simulink model "SimBAlink_CL"  (R2017a)
settings: Solver=ode1  StartTime=0.0  StopTime=Inf  FixedStep=0.01  RelTol=1e-3  EnableMultiTasking=on
PreLoadFcn:
  | clear all
  | close all
  | clc
  | 
  | currentFolder = pwd;
  | addpath(genpath(currentFolder));
values from neighbouring files (symbols this model uses):
  ambTemp_K = ambTemp_C + 273.5    [Initialize_Environment.m]    (also in Initialize_Environment_CDTS.m; Initialize_Environment_combined.m)
  Stoptime = 60    [Initialize_Environment.m]    (also in Initialize_Environment_CDTS.m; Initialize_Environment_combined.m; Initialize_Sim.m)
undefined symbols (not defined in the file or in its folder): BATT_ELEC, BATT_OCV, BATT_THERMAL, EM, MC, soc0
libraries: simulink x5
settings Model: Creator=bring  LastModifiedBy=bring
settings DataIOCC: LimitDataPoints=on  SaveFormat=Array  SignalLoggingSaveFormat=ModelDataLogs
settings OptimizationCC: ExpressionDepthLimit=2147483647  LifeSpan=inf
settings DebuggingCC: CheckSSInitialOutputMsg=off  UnderspecifiedInitializationDetection=Classic  MergeDetectMultiDrivingBlocksExec=none  SolverPrmCheckMsg=warning  FcnCallInpInsideContextMsg=warning  StateNameClashWarn=warning  SFUnexpectedBacktrackingDiag=warning  SFNoUnconditionalDefaultTransitionDiag=warning  SFExecutionAtInitializationDiag=none
settings HardwareCC: ProdBitPerPointer=32  ProdBitPerSizeT=32  ProdBitPerPtrDiffT=32  ProdLargestAtomicFloat=None  ProdIntDivRoundTo=Undefined  ProdEndianess=Unspecified  ProdWordSize=32  ProdHWDeviceType=32-bit Generic
settings ModelReferenceCC: PropagateSignalLabelsOutOfModel=off
settings SFSimCC: SimParseCustomCode=off
settings GRTTargetCC: TargetLangStandard=C89/C90 (ANSI)  GeneratePreprocessorConditionals=Disable all  CombineOutputUpdateFcns=off  GRTInterface=on
settings ConfigComp: CovMetricSettings=dw  CovHtmlReporting=on  CovSaveCumulativeToWorkspaceVar=on  CovSaveSingleToWorkspaceVar=on  CovExternalEMLEnable=off  CovSFcnEnable=off

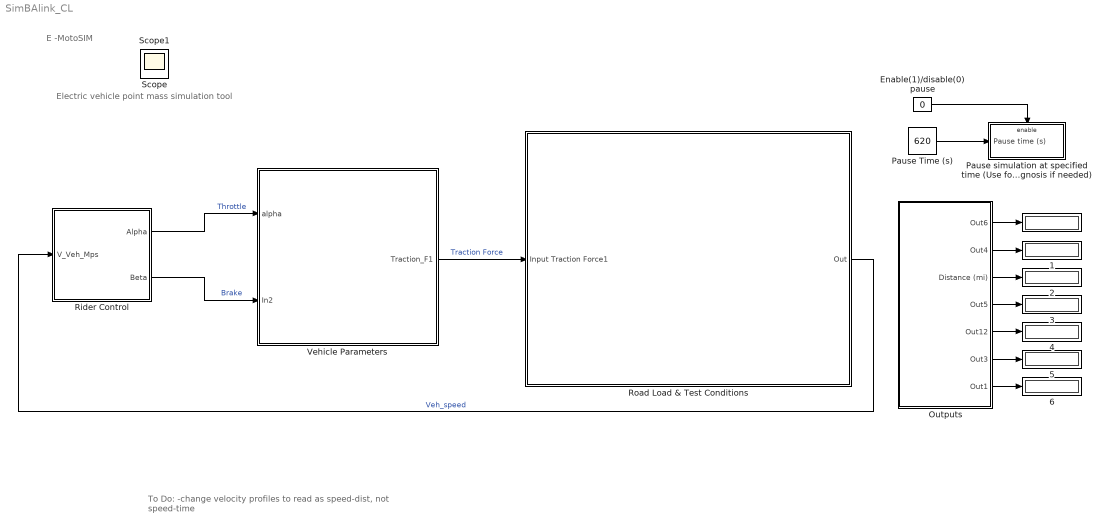
== system SimBAlink_CL ==
  note: To Do:
      | -change velocity profiles to read as speed-dist, not speed-time
  note: Electric vehicle point mass simulation tool
  note: E -MotoSIM
   {,1..6} (7 alike) : Display
  Enable(1)/disable(0) pause : Constant  Value=0
  Outputs : Subsystem  mask(Outputs){}
  Pause Time (s) : Constant  Value=620
  Pause simulation at specified time (Use for diagnosis if needed) : Subsystem
  Rider Control : Subsystem  mask(Driver){kp=1, ki=0.1, kd=0.1}
      mask prompts: kp "Proportional Gain"; ki "Integral Gain"; kd "Derivative Gain"
      mask help: Please select the PID controller gains to improve the tracking response.
      mask Display: image(imread('Images/helmet.jpg'))
  Road Load & Test Conditions : Subsystem  mask(Simulation Setup Options){DRIV_Cycle=US06_Highway_Cycle, rowA=1.13, ambTemp_C=20, soc0=95, Grade_Value=0, Wind_Speed=0, iteration=2, DRIV_acc_flag=off, DRIV_acc_final_v=100}
      mask prompts: DRIV_Cycle "Velocity Profile"; rowA "Air Density (kg.m^3)"; ambTemp_C "Ambient Temperature (C)"; soc0 "Battery Initial SOC (%)"; Grade_Value "Road Grade Climb (deg)"; Wind_Speed "Wind Speed (m/s)"; iteration "Driving Cycle Repetition"; DRIV_acc_flag "Acceleration Test"; DRIV_acc_final_v "Acceleration Test Final Velocity (mph)"
      mask init:
      | Initialize_Environment
      mask TypeOptions DRIV_Cycle: FHDS | FUDS | FUDS_fast | WLTP | US06 | US06_City_Cycle | US06_Highway_Cycle | Artemis_urban | Artemis_extra_urban | Artemis_highway | NEDC | PPIHC_CDTS
      mask Display: image(imread('images/bike.jpg'))
  Vehicle Parameters : Subsystem  mask(Vehicle Setup Options){baseMass=100, TIRE_radius=0.3, CdA=0.38, maxBrakeTorque=2000, FrontSprocket_toothCt=22, RearSprocket_toothCt=54, EM_MC_Selection=emrax268_PM150DZR, regenPct=0, CELL_Selection=LiFePo4_generic, cellSeriesCount=134, cellParallelCount=7, cellCapacity=17.5, ambTemp_C=270}
      mask prompts: baseMass "Vehicle+Rider Base Mass (kg)"; TIRE_radius "Tire Radius (m)"; maxBrakeTorque "Max Brake Torque (Nm)"; FrontSprocket_toothCt "Fr Sprocket Teeth"; RearSprocket_toothCt "Rr Sprocket Teeth"; EM_MC_Selection "Motor-MC Combo"; regenPct "Regen %"; CELL_Selection "Battery Cell Chemistry"; cellSeriesCount "Series Cells"; cellParallelCount "Parallel Cells"; cellCapacity "Cell Capacity (Ah)"; ambTemp_C "Ambient Temperature (C)"
      mask init:
      | Initialize_Vehicle
      mask TypeOptions EM_MC_Selection: emrax268_PM150DZR | ME708_KDS48200e
      mask TypeOptions CELL_Selection: LiFePo4_generic | A123_ANR26650
      mask DialogControl baseMass Tooltip: Vehicle+Rider Base Mass includes all components except EM, MC, and battery pack
      mask Display: image(imread('images/bike_powertrain.jpg'))
  Scope : Scope
  Scope1 : Scope
  wires:
  Road Load & Test Conditions/1(Out) -> Rider Control/1(V_Veh_Mps)  "Veh_speed"
  Rider Control/2(Beta) -> Vehicle Parameters/2(In2)  "Brake"
  Rider Control/1(Alpha) -> Vehicle Parameters/1(alpha)  "Throttle"
  Vehicle Parameters/1(Traction_F1) -> Road Load & Test Conditions/1(Input Traction Force1)  "Traction Force"
  Pause Time (s)/1 -> Pause simulation at specified time (Use for diagnosis if needed)/1(Pause time (s))
  Enable(1)/disable(0) pause/1 -> Pause simulation at specified time (Use for diagnosis if needed)/Enable
  Outputs/7(Out1) -> " 6"/1
  Outputs/6(Out3) -> " 5"/1
  Outputs/5(Out12) -> " 4"/1
  Outputs/4(Out5) -> " 3"/1
  Outputs/3(Distance (mi)) -> " 2"/1
  Outputs/2(Out4) -> " 1"/1
  Outputs/1(Out6) -> " "/1

== system SimBAlink_CL/Outputs ==
  Battery Outputs : Subsystem
  Driver : Subsystem
  EM Outputs : Subsystem
  Vehicle Parameters : Subsystem
  Out6 : Outport
  Out4 : Outport  Port=2
  Distance (mi) : Outport  Port=3
  Out5 : Outport  Port=4
  Out12 : Outport  Port=5
  Out3 : Outport  Port=6
  Out1 : Outport  Port=7
  wires:
  Battery Outputs/3(Out2) -> Distance (mi)/1
  Battery Outputs/1(Out5) -> Out5/1
  EM Outputs/1(Out7) -> Out3/1
  EM Outputs/2(Out8) -> Out1/1
  Vehicle Parameters/1(Distance (mi)) -> Out4/1  "Distance (mi)"
  Vehicle Parameters/2(Out2) -> Out6/1
  Battery Outputs/2(Out1) -> Out12/1

== system SimBAlink_CL/Pause simulation at specified time (Use for diagnosis if needed) ==
  Pause time (s) : Inport
  Enable : EnablePort
  Add1 : Sum  Inputs=+-
  Assertion1 : Assertion  AssertionFailFcn=|  StopWhenAssertionFail=off
      | set_param(bdroot,'SimulationCommand','pause'),
      | disp(sprintf('\nSimulation paused.'))
  Clock1 : Clock
  Compare To Zero1 : simulink/Logic and Bit Operations/Compare To Zero  relop=~=  OutDataTypeStr=boolean
  wires:
  Clock1/1 -> Add1/1
  Compare To Zero1/1 -> Assertion1/1
  Add1/1 -> Compare To Zero1/1
  Pause time (s)/1 -> Add1/2

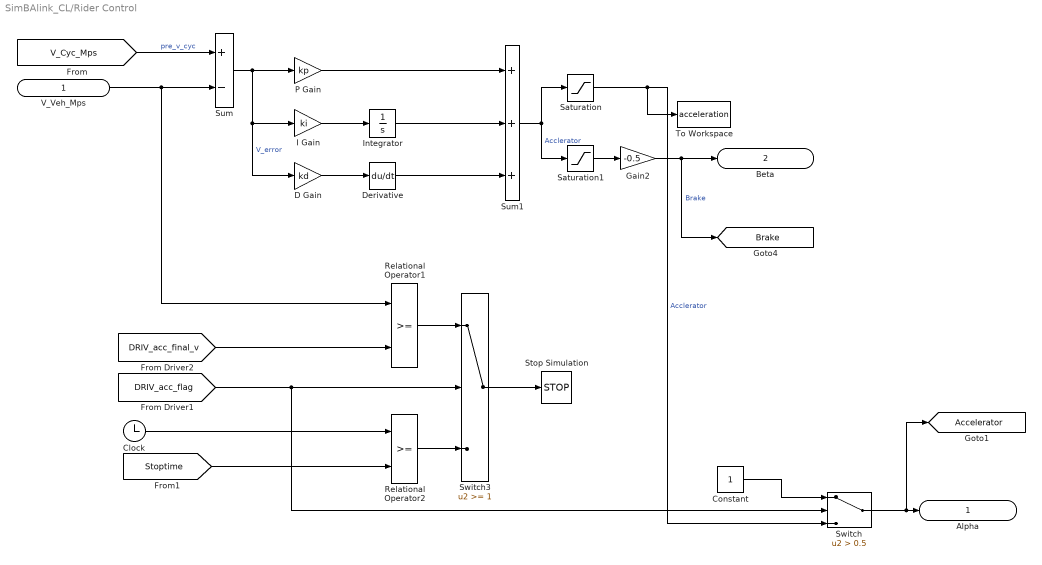
== system SimBAlink_CL/Rider Control ==
  V_Veh_Mps : Inport
  Clock : Clock
  Constant : Constant
  D Gain : Gain  Gain=kd
  Derivative : Derivative
  Gain2 : Gain  Gain=-0.5
  I Gain : Gain  Gain=ki
  Integrator : Integrator  UpperSaturationLimit=0.4
  P Gain : Gain  Gain=kp
  Relational Operator1 : RelationalOperator  RndMeth=Nearest  InputSameDT=on
  Relational Operator2 : RelationalOperator  RndMeth=Nearest  InputSameDT=on
  Saturation : Saturate  UpperLimit=1  LowerLimit=0
  Saturation1 : Saturate  UpperLimit=0  LowerLimit=-1
  Stop Simulation : Stop
  Sum : Sum  Inputs=+-
  Sum1 : Sum  Inputs=+++
  Switch : Switch  Criteria=u2 > Threshold  Threshold=0.5
  Switch3 : Switch  Threshold=1  SaturateOnIntegerOverflow=on  InputSameDT=on
  To Workspace : ToWorkspace  VariableName=acceleration  SampleTime=-1
  Alpha : Outport
  Beta : Outport  Port=2
  tag scope: Accelerator=global, Brake=global
  wires:
  Gain2/1 -> [Brake], Beta/1  "Brake"
  Sum1/1 -> Saturation/1, Saturation1/1  "Acclerator"
  D Gain/1 -> Derivative/1
  I Gain/1 -> Integrator/1
  Saturation/1 -> To Workspace/1, Switch/3  "Acclerator"
  Saturation1/1 -> Gain2/1
  Clock/1 -> Relational Operator2/1
  [Stoptime] -> Relational Operator2/2
  [DRIV_acc_flag] -> Switch/2, Switch3/2
  Relational Operator1/1 -> Switch3/1
  [DRIV_acc_final_v] -> Relational Operator1/2
  Switch3/1 -> Stop Simulation/1
  Relational Operator2/1 -> Switch3/3
  Constant/1 -> Switch/1
  Switch/1 -> [Accelerator], Alpha/1
  Derivative/1 -> Sum1/3
  Integrator/1 -> Sum1/2
  P Gain/1 -> Sum1/1
  [V_Cyc_Mps] -> Sum/1  "pre_v_cyc"
  Sum/1 -> P Gain/1, D Gain/1, I Gain/1  "V_error"
  V_Veh_Mps/1 -> Relational Operator1/1, Sum/2

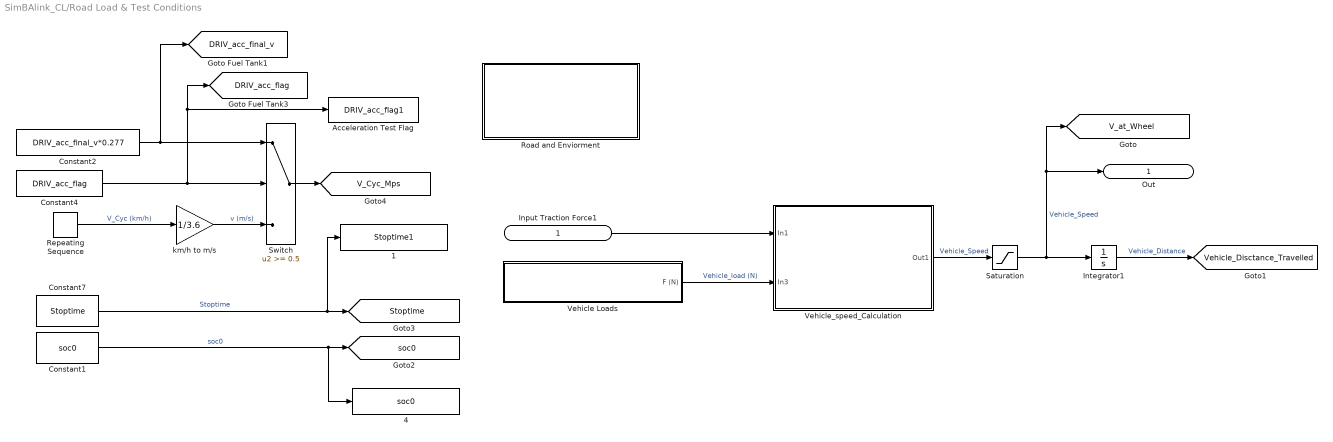
== system SimBAlink_CL/Road Load & Test Conditions ==
  Input Traction Force1 : Inport
  " 1" : ToWorkspace  VariableName=Stoptime1  SampleTime=-1
      settings: MaxDataPoints=1
  " 4" : ToWorkspace  VariableName=soc0  SampleTime=-1
      settings: MaxDataPoints=1
  Acceleration Test Flag : ToWorkspace  VariableName=DRIV_acc_flag1  SampleTime=-1
  Constant1 : Constant  Value=soc0
  Constant2 : Constant  Value=DRIV_acc_final_v*0.277
  Constant4 : Constant  Value=DRIV_acc_flag
  Constant7 : Constant  Value=Stoptime
  Integrator1 : Integrator
  Repeating Sequence : simulink/Sources/Repeating Sequence  rep_seq_t=t_cyc  rep_seq_y=v_cyc
  Road and Enviorment : Subsystem
      mask Display: text(.5,.5,'\fontsize{10}{ Road and Environment}', 'hor','center','texmode','on');
  Saturation : Saturate  UpperLimit=inf  LowerLimit=0
  Switch : Switch  Threshold=0.5
  Vehicle Loads : Subsystem
  Vehicle_speed_Calculation : Subsystem
  km/h to m/s : Gain  Gain=1/3.6
  Out : Outport
  tag scope: DRIV_acc_final_v=global, DRIV_acc_flag=global, Stoptime=global, V_Cyc_Mps=global, V_at_Wheel=global, Vehicle_Disctance_Travelled=global, soc0=global
  wires:
  Vehicle Loads/1(F (N)) -> Vehicle_speed_Calculation/2(In3)  "Vehicle_load (N)"
  Input Traction Force1/1 -> Vehicle_speed_Calculation/1(In1)
  Vehicle_speed_Calculation/1(Out1) -> Saturation/1  "Vehicle_Speed"
  Integrator1/1 -> [Vehicle_Disctance_Travelled]  "Vehicle_Distance"
  Saturation/1 -> Out/1, [V_at_Wheel], Integrator1/1  "Vehicle_Speed"
  Constant1/1 -> [soc0], " 4"/1  "soc0"
  Repeating Sequence/1 -> km/h to m/s/1  "V_Cyc (km/h)"
  Constant7/1 -> [Stoptime], " 1"/1  "Stoptime"
  Constant4/1 -> Switch/2, [DRIV_acc_flag], Acceleration Test Flag/1
  Switch/1 -> [V_Cyc_Mps]
  km/h to m/s/1 -> Switch/3  "v (m/s)"
  Constant2/1 -> Switch/1, [DRIV_acc_final_v]

== system SimBAlink_CL/Vehicle Parameters ==
  alpha : Inport
  In2 : Inport  Port=2
  Battery Pack : Subsystem
      mask Display: image(imread('Images/pack.jpg'))
  Electric Motor and Motor Controller : Subsystem
      mask Display: image(imread('Images/idu.jpg'))
  Final Drive : Subsystem
      mask Display: image(imread('Images/gear.jpg'))
  Powertrain Controller : Subsystem
  Sum1 : Sum  Inputs=+|+
  Vehicle Brakes Front : Subsystem  mask(Brake){Brake_Position=[0 .14 0.31 0.46 0.76 1], Brake_Torque=[0 90.3 180.95 270.83 4600.4 6100]}
      mask prompts: Brake_Position "Brake Position"; Brake_Torque "Brake Torque"
      mask help:
      | This block calculates the brake torque using a 1D map between Brake position and Brake Torque
      | The inputs are the Brake Position array between 0 and 1 and the respective Brake Torque values.
      mask Display: image(imread('images/motoBrake.jpg'))
  Vehicle Brakes Rear : Subsystem  mask(Brake){Brake_Position=[0 .14 0.31 0.46 0.76 1], Brake_Torque=[0 90.3 180.95 270.83 4600.4 6100]}
      mask prompts: Brake_Position "Brake Position"; Brake_Torque "Brake Torque"
      mask help:
      | This block calculates the brake torque using a 1D map between Brake position and Brake Torque
      | The inputs are the Brake Position array between 0 and 1 and the respective Brake Torque values.
      mask Display: image(imread('images/motoBrake.jpg'))
  Vehicle Front Wheels : Subsystem
      mask Display: image(imread('Images/frTire_pirelli.jpg'))
  Vehicle Parameters : Subsystem
      mask Display: text(.5,.5,'\fontsize{10}{Vehicle Parameters}', 'hor','center','texmode','on');
  Vehicle Rear Wheels : Subsystem
      mask Display: image(imread('Images/rrTire_pirelli.jpg'))
  Traction_F1 : Outport
  wires:
  Vehicle Brakes Front/1(Out1) -> Vehicle Front Wheels/1(In1)
  alpha/1 -> Powertrain Controller/1(alpha)
  Vehicle Brakes Rear/1(Out1) -> Vehicle Rear Wheels/1(In1)
  In2/1 -> Powertrain Controller/2(In2)
  Powertrain Controller/3(Engine_Torque_Request) -> Vehicle Brakes Rear/2(Beta (Braking))
  Powertrain Controller/1(Engine_Torque_Request3) -> Vehicle Brakes Front/1(Beta (Braking))
  Electric Motor and Motor Controller/2(EM_RPM) -> Final Drive/1(Torque EM)
  Final Drive/1(EM Torque) -> Vehicle Brakes Rear/1(Torque_out_REM_gearbox)
  Sum1/1 -> Traction_F1/1  "Traction Force"
  Vehicle Front Wheels/1(Out1) -> Sum1/1  "Front Traction Force"
  Vehicle Rear Wheels/1(Out1) -> Sum1/2  "Rear Traction Force"
  Powertrain Controller/2(Engine_Torque_Request4) -> Electric Motor and Motor Controller/1(Torque EM)
  Electric Motor and Motor Controller/1(MC_request_Pwr) -> Battery Pack/1(MC_request_Pwr)

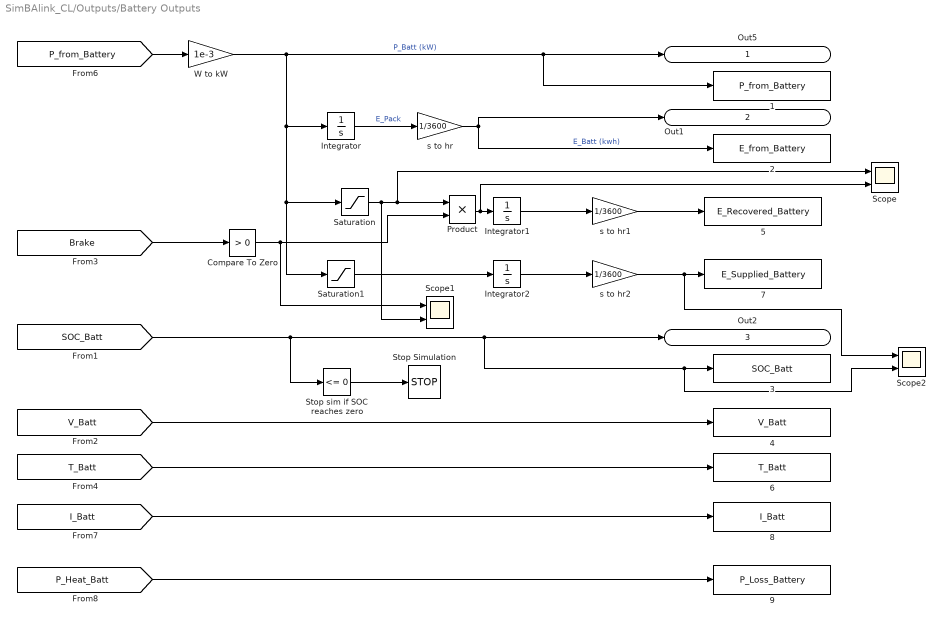
== system SimBAlink_CL/Outputs/Battery Outputs ==
  " 1" : ToWorkspace  VariableName=P_from_Battery  SampleTime=-1
  " 2" : ToWorkspace  VariableName=E_from_Battery  SampleTime=-1
  " 3" : ToWorkspace  VariableName=SOC_Batt  SampleTime=-1
  " 4" : ToWorkspace  VariableName=V_Batt  SampleTime=-1
  " 5" : ToWorkspace  VariableName=E_Recovered_Battery  SampleTime=-1
  " 6" : ToWorkspace  VariableName=T_Batt  SampleTime=-1
  " 7" : ToWorkspace  VariableName=E_Supplied_Battery  SampleTime=-1
  " 8" : ToWorkspace  VariableName=I_Batt  SampleTime=-1
  " 9" : ToWorkspace  VariableName=P_Loss_Battery  SampleTime=-1
  Compare To Zero : simulink/Logic and Bit Operations/Compare To Zero  relop=>  OutDataTypeStr=boolean
  Integrator : Integrator
  Integrator1 : Integrator
  Integrator2 : Integrator
  Product : Product  RndMeth=Zero
  Saturation : Saturate  UpperLimit=0  LowerLimit=-inf
  Saturation1 : Saturate  UpperLimit=inf  LowerLimit=0
  Scope : Scope  NumInputPorts=2
  Scope1 : Scope  NumInputPorts=2
  Scope2 : Scope  NumInputPorts=2
  Stop Simulation : Stop
  Stop sim if SOC reaches zero : simulink/Logic and Bit Operations/Compare To Zero  relop=<=  OutDataTypeStr=boolean
  W to kW : Gain  Gain=1e-3
  s to hr : Gain  Gain=1/3600
  s to hr1 : Gain  Gain=1/3600
  s to hr2 : Gain  Gain=1/3600
  Out5 : Outport
  Out1 : Outport  Port=2
  Out2 : Outport  Port=3
  wires:
  [P_from_Battery] -> W to kW/1
  Integrator/1 -> s to hr/1  "E_Pack"
  [SOC_Batt] -> Stop sim if SOC reaches zero/1, Out2/1, Scope2/2, " 3"/1
  [V_Batt] -> " 4"/1
  [I_Batt] -> " 8"/1
  [P_Heat_Batt] -> " 9"/1
  s to hr/1 -> Out1/1, " 2"/1  "E_Batt (kwh)"
  s to hr1/1 -> " 5"/1
  Integrator1/1 -> s to hr1/1
  W to kW/1 -> Out5/1, " 1"/1, Integrator/1, Saturation1/1, Saturation/1  "P_Batt (kW)"
  s to hr2/1 -> Scope2/1, " 7"/1
  Integrator2/1 -> s to hr2/1
  Saturation1/1 -> Integrator2/1
  [Brake] -> Compare To Zero/1
  Product/1 -> Scope/2, Integrator1/1
  Saturation/1 -> Scope1/2, Scope/1, Product/1
  Compare To Zero/1 -> Scope1/1, Product/2
  [T_Batt] -> " 6"/1
  Stop sim if SOC reaches zero/1 -> Stop Simulation/1

== system SimBAlink_CL/Outputs/Driver ==
  To Workspace1 : ToWorkspace  VariableName=Brake_pedal  SampleTime=-1
  To Workspace6 : ToWorkspace  VariableName=Acc_pedal  SampleTime=-1
  wires:
  [Brake] -> To Workspace1/1
  [Accelerator] -> To Workspace6/1

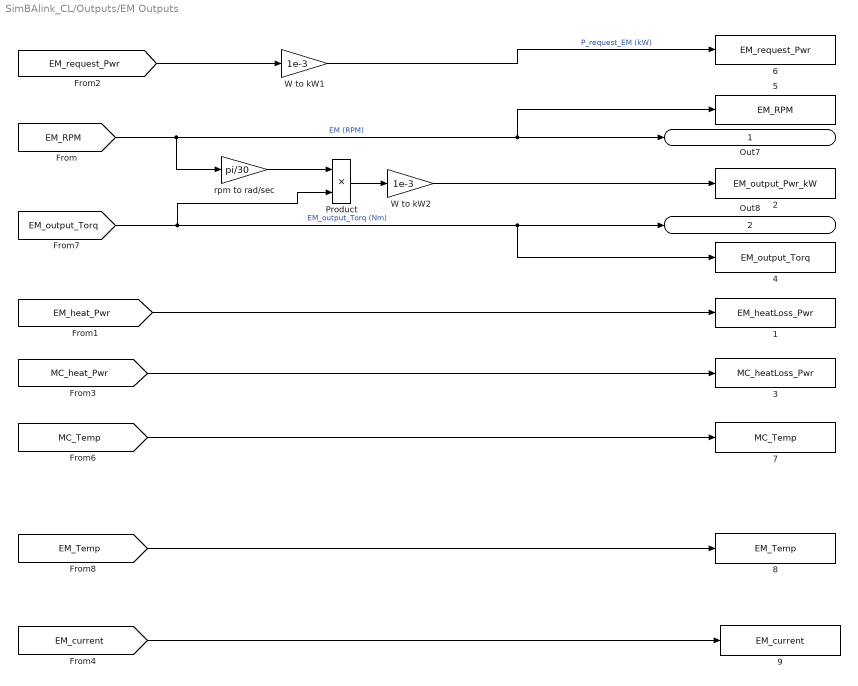
== system SimBAlink_CL/Outputs/EM Outputs ==
  " 1" : ToWorkspace  VariableName=EM_heatLoss_Pwr  SampleTime=-1
  " 2" : ToWorkspace  VariableName=EM_output_Pwr_kW  SampleTime=-1
  " 3" : ToWorkspace  VariableName=MC_heatLoss_Pwr  SampleTime=-1
  " 4" : ToWorkspace  VariableName=EM_output_Torq  SampleTime=-1
  " 5" : ToWorkspace  VariableName=EM_RPM  SampleTime=-1
  " 6" : ToWorkspace  VariableName=EM_request_Pwr  SampleTime=-1
  " 7" : ToWorkspace  VariableName=MC_Temp  SampleTime=-1
  " 8" : ToWorkspace  VariableName=EM_Temp  SampleTime=-1
  " 9" : ToWorkspace  VariableName=EM_current  SampleTime=-1
  Product : Product
  W to kW1 : Gain  Gain=1e-3
  W to kW2 : Gain  Gain=1e-3
  rpm to rad/sec : Gain  Gain=pi/30
  Out7 : Outport
  Out8 : Outport  Port=2
  wires:
  [EM_output_Torq] -> Product/2, " 4"/1, Out8/1  "EM_output_Torq (Nm)"
  [EM_RPM] -> " 5"/1, Out7/1, rpm to rad/sec/1  "EM (RPM)"
  W to kW1/1 -> " 6"/1  "P_request_EM (kW)"
  [EM_request_Pwr] -> W to kW1/1
  Product/1 -> W to kW2/1
  W to kW2/1 -> " 2"/1
  rpm to rad/sec/1 -> Product/1
  [MC_heat_Pwr] -> " 3"/1
  [EM_heat_Pwr] -> " 1"/1
  [EM_Temp] -> " 8"/1
  [MC_Temp] -> " 7"/1
  [EM_current] -> " 9"/1

== system SimBAlink_CL/Outputs/Vehicle Parameters ==
  " " : ToWorkspace  VariableName=T_simulation  SampleTime=-1
  " 1" : ToWorkspace  VariableName=mode  SampleTime=-1
  Clock : Clock
  To Workspace5 : ToWorkspace  VariableName=Desired_Speed_mph  SampleTime=-1
  To Workspace6 : ToWorkspace  VariableName=Vehicle_Speed_mph  SampleTime=-1
  m to mi : Gain  Gain=0.000621371
  m/s to mph : Gain  Gain=2.237
  m/s to mph1 : Gain  Gain=2.237
  Distance (mi) : Outport
  Out2 : Outport  Port=2
  wires:
  [Vehicle_Disctance_Travelled] -> m to mi/1
  m to mi/1 -> Distance (mi)/1  "Distance (mi)"
  [V_Cyc_Mps] -> m/s to mph/1
  [V_at_Wheel] -> m/s to mph1/1
  m/s to mph/1 -> To Workspace5/1
  Clock/1 -> " "/1, Out2/1  "Time (sec)"
  m/s to mph1/1 -> To Workspace6/1
  [Mode] -> " 1"/1  "Mode"

== system SimBAlink_CL/Road Load & Test Conditions/Road and Enviorment ==
  Constant1 : Constant  Value=Wind_Speed
  Constant2 : Constant  Value=ambTemp_K
  Constant3 : Constant  Value=ambTemp_C
  Constant4 : Constant  Value=rowA
  Constant5 : Constant  Value=Grade_Value
  tag scope: Road_Grade=global, Row_Air=global, Wind_Speed=global, ambTemp_C=global, ambTemp_K=global
  wires:
  Constant4/1 -> [Row_Air]  "air density"
  Constant5/1 -> [Road_Grade]  "road grade"
  Constant1/1 -> [Wind_Speed]  "wind speed"
  Constant2/1 -> [ambTemp_K]
  Constant3/1 -> [ambTemp_C]

== system SimBAlink_CL/Road Load & Test Conditions/Vehicle Loads ==
  Aerodynamic  Drag : Subsystem
  Display1 : Display
      settings: Decimation=5
  Display2 : Display
      settings: Decimation=5
  Display3 : Display
      settings: Decimation=5
  Grade Force : Subsystem
  Roll Force : Subsystem
  Sum4 : Sum  Inputs=+++
  F (N) : Outport
  wires:
  Sum4/1 -> F (N)/1  "Road Load (N)"
  Roll Force/1(Power_roll) -> Display3/1, Sum4/3
  Aerodynamic  Drag/1(Drag Power) -> Display1/1, Sum4/2
  Grade Force/1(Drag Power) -> Display2/1, Sum4/1

== system SimBAlink_CL/Road Load & Test Conditions/Vehicle_speed_Calculation ==
  In1 : Inport
  In3 : Inport  Port=2
  Display : Display
  Display1 : Display
  Divide : Product  Inputs=*//
  Integrator : Integrator  InitialCondition=0.0001  LimitOutput=on  LowerSaturationLimit=0
  Mass factor : Constant  Value=1.0
  Sum : Sum  Inputs=+-
  Out1 : Outport
  wires:
  Sum/1 -> Divide/1  "Net_Force"
  Divide/1 -> Integrator/1  "Vehicle_Acceleration"
  In1/1 -> Display/1, Sum/1
  Integrator/1 -> Out1/1  "Vehicle_Speed"
  [M] -> Divide/2
  In3/1 -> Display1/1, Sum/2
  Mass factor/1 -> Divide/3

== system SimBAlink_CL/Vehicle Parameters/Battery Pack ==
  MC_request_Pwr : Inport
  Battery Parameters Calculation : Subsystem
      mask Display:
      | color('blue');
      | fprintf('Battery Parameters Calculation')
  Battery to Cell : Subsystem
      mask Display:
      | color('blue');
      | fprintf('Battery to Cell')
  Cell : Subsystem
      mask Display:
      | color('blue');
      | fprintf('Cell: 1st Order Electrical Model')
  Cell to Batt : Subsystem
      mask Display:
      | color('blue');
      | fprintf('Cell to Battery')
  Current Limiter : Saturate  UpperLimit=180  LowerLimit=-60
  Divide : Product  Inputs=/*
  Memory : Memory
  Sum : Sum
  Thermal Dynamics : Subsystem
      mask Display:
      | color('blue');
      | fprintf('Battery Thermal')
  tag scope: P_from_Battery=global
  wires:
  Divide/1 -> Memory/1  "I_Batt_Req"
  Battery to Cell/1(Out1) -> Cell/1(In2)
  Cell/1(Out1) -> Cell to Batt/1(In1)
  Cell/2(Out2) -> Cell to Batt/2(In2)
  Cell to Batt/1(Out1) -> Divide/1
  Current Limiter/1 -> Battery Parameters Calculation/1(current1), Battery to Cell/1(In1)  "I_Batt"
  Cell to Batt/2(Out3) -> [P_from_Battery]
  Memory/1 -> Current Limiter/1
  [P_Heat_Batt] -> Sum/1
  Sum/1 -> Divide/2  "P_Req"
  MC_request_Pwr/1 -> Sum/2  "MC_request_Pwr"

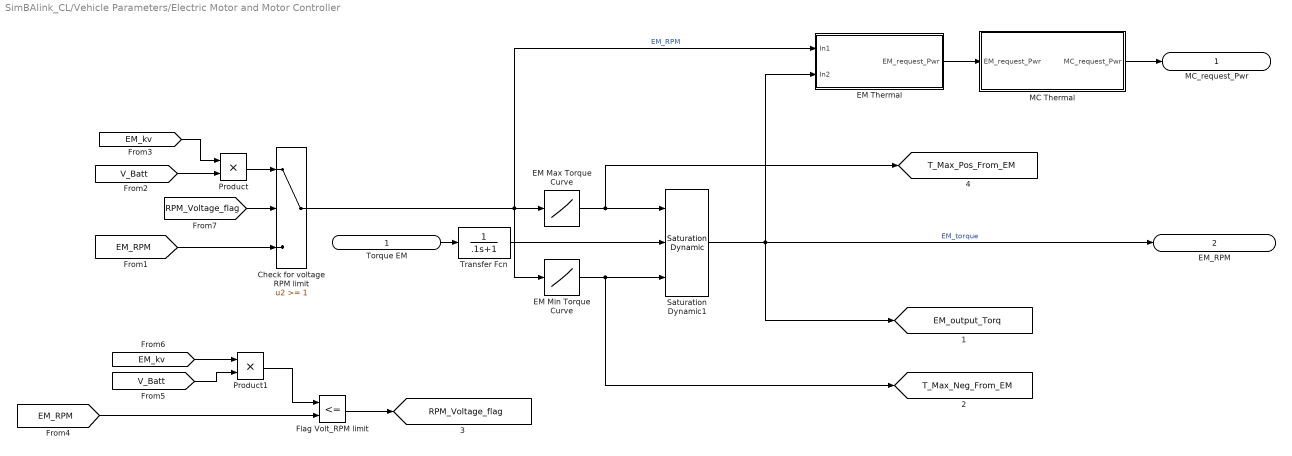
== system SimBAlink_CL/Vehicle Parameters/Electric Motor and Motor Controller ==
  Torque EM : Inport
  Check for voltage RPM limit : Switch  Threshold=1  SaturateOnIntegerOverflow=on  InputSameDT=on
  EM Max Torque Curve : Lookup  InputValues=EM.N_RPM  Table=EM.T_max_Peak  LookUpMeth=Interpolation-Use End Values  SaturateOnIntegerOverflow=on
  EM Min Torque Curve : Lookup  InputValues=EM.N_RPM  Table=EM.T_min_Peak  LookUpMeth=Interpolation-Use End Values  SaturateOnIntegerOverflow=on
  EM Thermal : Subsystem
  Flag Volt_RPM limit : RelationalOperator  Operator=<=  OutDataTypeStr=boolean  RndMeth=Simplest
  MC Thermal : Subsystem
  Product : Product
  Product1 : Product
  Saturation Dynamic1 : simulink/Discontinuities/Saturation Dynamic  OutMin=[]  OutMax=[]  OutDataTypeStr=Inherit: Same as second input  OutDataType=sfix(16)  OutScaling=2^-10  DoSatur=off
  Transfer Fcn : TransferFcn  Denominator=[.1 1]
  MC_request_Pwr : Outport
  EM_RPM : Outport  Port=2
  tag scope: EM_output_Torq=global, RPM_Voltage_flag=global, T_Max_Neg_From_EM=global, T_Max_Pos_From_EM=global
  wires:
  Check for voltage RPM limit/1 -> EM Min Torque Curve/1, EM Thermal/1(In1), EM Max Torque Curve/1  "EM_RPM"
  EM Max Torque Curve/1 -> Saturation Dynamic1/1, [T_Max_Pos_From_EM]
  EM Min Torque Curve/1 -> Saturation Dynamic1/3, [T_Max_Neg_From_EM]
  Torque EM/1 -> Transfer Fcn/1
  Saturation Dynamic1/1 -> [EM_output_Torq], EM Thermal/2(In2), EM_RPM/1  "EM_torque"
  Transfer Fcn/1 -> Saturation Dynamic1/2
  EM Thermal/1(EM_request_Pwr) -> MC Thermal/1(EM_request_Pwr)
  MC Thermal/1(MC_request_Pwr) -> MC_request_Pwr/1
  [V_Batt] -> Product/2
  [EM_kv] -> Product/1
  Product/1 -> Check for voltage RPM limit/1
  [EM_RPM] -> Check for voltage RPM limit/3
  [EM_RPM] -> Flag Volt_RPM limit/2
  Product1/1 -> Flag Volt_RPM limit/1
  [EM_kv] -> Product1/1
  [V_Batt] -> Product1/2
  Flag Volt_RPM limit/1 -> [RPM_Voltage_flag]
  [RPM_Voltage_flag] -> Check for voltage RPM limit/2

== system SimBAlink_CL/Vehicle Parameters/Final Drive ==
  Torque EM : Inport
  "CONVERT TO whl RPM " : Gain  Gain=60
  Calc wheel circumference : Gain  Gain=2*3.14
  Display : Display
  "convert to whl rev per sec " : Product  Inputs=*/
  "product rpm " : Product  Inputs=**
  product rpm 1 : Product  Inputs=***
  EM Torque : Outport
  tag scope: EM_RPM=global
  wires:
  [V_at_Wheel] -> "convert to whl rev per sec "/1
  "convert to whl rev per sec "/1 -> "CONVERT TO whl RPM "/1
  product rpm 1/1 -> EM Torque/1  "Torque_out_EM_gearbox"
  [Rr_Wheel_Radius] -> Calc wheel circumference/1
  Calc wheel circumference/1 -> "convert to whl rev per sec "/2
  "CONVERT TO whl RPM "/1 -> "product rpm "/1
  "product rpm "/1 -> [EM_RPM]
  [Final_Drive_Ratio] -> Display/1, "product rpm "/2, product rpm 1/1
  [Final_Drive_Eff] -> product rpm 1/3
  Torque EM/1 -> product rpm 1/2

== system SimBAlink_CL/Vehicle Parameters/Powertrain Controller ==
  alpha : Inport
  In2 : Inport  Port=2
  Braking Strategy : Subsystem
  Constant : Constant
  Constant1 : Constant  Value=4
  Memory2 : Memory
  Switch1 : Switch  Criteria=u2 > Threshold  Threshold=0.01
  Switch2 : Switch  Criteria=u2 > Threshold
  Traction Torque Strategy : Subsystem
  Engine_Torque_Request3 : Outport
  Engine_Torque_Request4 : Outport  Port=2
  Engine_Torque_Request : Outport  Port=3
  tag scope: Mode=global
  wires:
  Braking Strategy/2(Out2) -> Engine_Torque_Request/1
  In2/1 -> Braking Strategy/1(In1)
  Braking Strategy/3(Out3) -> Engine_Torque_Request3/1
  Switch1/1 -> Memory2/1  "REM_T_Request"
  alpha/1 -> Switch2/2, Switch1/2, Traction Torque Strategy/1(In1)
  Traction Torque Strategy/1(REM_Torque_Request) -> Switch1/1
  Braking Strategy/1(Out4) -> Switch1/3
  Memory2/1 -> Engine_Torque_Request4/1
  Switch2/1 -> [Mode]
  Constant/1 -> Switch2/1
  Constant1/1 -> Switch2/3

== system SimBAlink_CL/Vehicle Parameters/Vehicle Brakes Front ==
  Beta (Braking) : Inport
  "ApplyNegForce " : Gain  Gain=-1
  Product : Product
  Out1 : Outport
  wires:
  Beta (Braking)/1 -> Product/1
  "ApplyNegForce "/1 -> Out1/1  "Net_Torque"
  Product/1 -> "ApplyNegForce "/1  "Net_Torque"
  [maxBrakeTorque] -> Product/2

== system SimBAlink_CL/Vehicle Parameters/Vehicle Brakes Rear ==
  Torque_out_REM_gearbox : Inport
  Beta (Braking) : Inport  Port=2
  Product : Product
  Sum : Sum  Inputs=-+  SaturateOnIntegerOverflow=on  InputSameDT=on  OutDataTypeStr=Inherit: Same as first input
  Out1 : Outport
  wires:
  Torque_out_REM_gearbox/1 -> Sum/2  "Torque_out_REM_gearbox"
  Sum/1 -> Out1/1  "Rear_Net_Torque"
  Product/1 -> Sum/1
  Beta (Braking)/1 -> Product/1
  [maxBrakeTorque] -> Product/2

== system SimBAlink_CL/Vehicle Parameters/Vehicle Front Wheels ==
  In1 : Inport
  Divide : Product  Inputs=*/
  Out1 : Outport
  wires:
  [Fr_Wheel_Radius] -> Divide/2
  In1/1 -> Divide/1
  Divide/1 -> Out1/1  "Tractive_Force_Front"

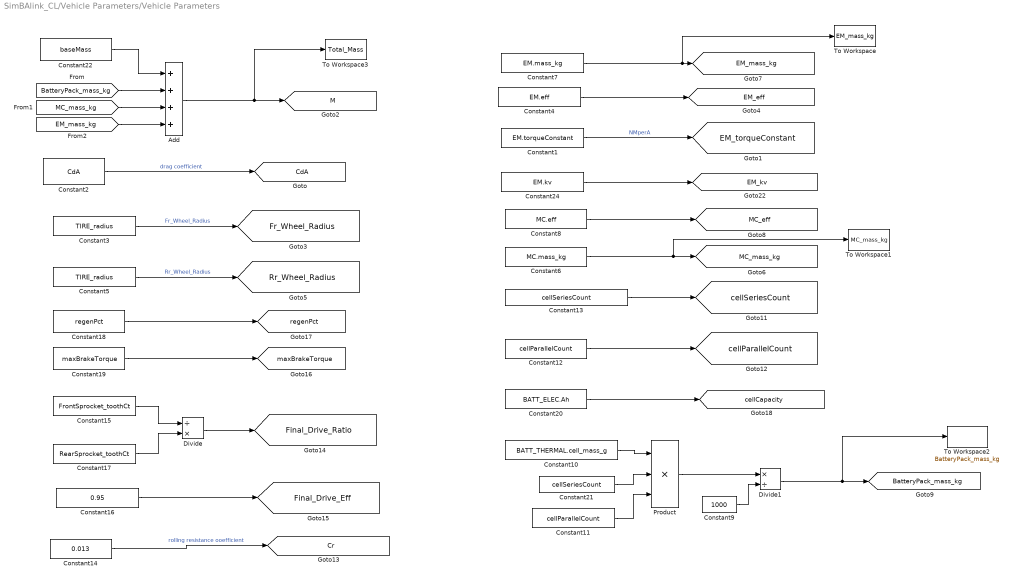
== system SimBAlink_CL/Vehicle Parameters/Vehicle Parameters ==
  Add : Sum  Inputs=++++
  Constant1 : Constant  Value=EM.torqueConstant
  Constant10 : Constant  Value=BATT_THERMAL.cell_mass_g
  Constant11 : Constant  Value=cellParallelCount
  Constant12 : Constant  Value=cellParallelCount
  Constant13 : Constant  Value=cellSeriesCount
  Constant14 : Constant  Value=0.013
  Constant15 : Constant  Value=FrontSprocket_toothCt
  Constant16 : Constant  Value=0.95
  Constant17 : Constant  Value=RearSprocket_toothCt
  Constant18 : Constant  Value=regenPct
  Constant19 : Constant  Value=maxBrakeTorque
  Constant2 : Constant  Value=CdA
  Constant20 : Constant  Value=BATT_ELEC.Ah
  Constant21 : Constant  Value=cellSeriesCount
  Constant22 : Constant  Value=baseMass
  Constant24 : Constant  Value=EM.kv
  Constant3 : Constant  Value=TIRE_radius
  Constant4 : Constant  Value=EM.eff
  Constant5 : Constant  Value=TIRE_radius
  Constant6 : Constant  Value=MC.mass_kg
  Constant7 : Constant  Value=EM.mass_kg
  Constant8 : Constant  Value=MC.eff
  Constant9 : Constant  Value=1000
  Divide : Product  Inputs=/*
  Divide1 : Product  Inputs=*/
  Product : Product  Inputs=3
  To Workspace : ToWorkspace  VariableName=EM_mass_kg  SaveFormat=Timeseries  SampleTime=-1
  To Workspace1 : ToWorkspace  VariableName=MC_mass_kg  SaveFormat=Timeseries  SampleTime=-1
  To Workspace2 : ToWorkspace  VariableName=BatteryPack_mass_kg  SaveFormat=Timeseries  SampleTime=-1
  To Workspace3 : ToWorkspace  VariableName=Total_Mass  SaveFormat=Timeseries  SampleTime=-1
  tag scope: BatteryPack_mass_kg=global, CdA=global, Cr=global, EM_eff=global, EM_kv=global, EM_mass_kg=global, EM_torqueConstant=global, Final_Drive_Eff=global, Final_Drive_Ratio=global, Fr_Wheel_Radius=global, M=global, MC_eff=global, MC_mass_kg=global, Rr_Wheel_Radius=global, cellCapacity=global, cellParallelCount=global, cellSeriesCount=global, maxBrakeTorque=global, regenPct=global
  wires:
  Constant2/1 -> [CdA]  "drag coefficient"
  Constant3/1 -> [Fr_Wheel_Radius]  "Fr_Wheel_Radius"
  Constant4/1 -> [EM_eff]
  Constant5/1 -> [Rr_Wheel_Radius]  "Rr_Wheel_Radius"
  Constant8/1 -> [MC_eff]
  Constant13/1 -> [cellSeriesCount]
  Constant12/1 -> [cellParallelCount]
  Constant14/1 -> [Cr]  "rolling resistance ooefficient"
  Constant1/1 -> [EM_torqueConstant]  "NMperA"
  Constant16/1 -> [Final_Drive_Eff]
  Constant15/1 -> Divide/1
  Divide/1 -> [Final_Drive_Ratio]
  Constant17/1 -> Divide/2
  Constant19/1 -> [maxBrakeTorque]
  Constant18/1 -> [regenPct]
  Constant20/1 -> [cellCapacity]
  Add/1 -> To Workspace3/1, [M]
  Constant24/1 -> [EM_kv]
  Constant6/1 -> To Workspace1/1, [MC_mass_kg]
  Constant7/1 -> To Workspace/1, [EM_mass_kg]
  Constant10/1 -> Product/1
  Constant21/1 -> Product/2
  Constant11/1 -> Product/3
  Constant22/1 -> Add/1
  [BatteryPack_mass_kg] -> Add/2
  [EM_mass_kg] -> Add/4
  [MC_mass_kg] -> Add/3
  Product/1 -> Divide1/1
  Divide1/1 -> To Workspace2/1, [BatteryPack_mass_kg]
  Constant9/1 -> Divide1/2

== system SimBAlink_CL/Vehicle Parameters/Vehicle Rear Wheels ==
  In1 : Inport
  Divide : Product  Inputs=*/
  Out1 : Outport
  wires:
  [Rr_Wheel_Radius] -> Divide/2
  In1/1 -> Divide/1
  Divide/1 -> Out1/1  "Tractive_Force_Rear"

== system SimBAlink_CL/Road Load & Test Conditions/Vehicle Loads/Aerodynamic  Drag ==
  Constant : Constant  Value=0.5
  Display : Display
      settings: Decimation=5
  Drag force =1/2*row_a*Cd*Af*v2 : Product  Inputs=4  RndMeth=Zero
  Sum : Sum  Inputs=|++
  drag_v1 : Math  Operator=pow  SaturateOnIntegerOverflow=on
  square : Constant  Value=2
  Drag Power : Outport
  wires:
  square/1 -> drag_v1/2
  Constant/1 -> Drag force =1/2*row_a*Cd*Af*v2/1
  [CdA] -> Drag force =1/2*row_a*Cd*Af*v2/3
  [Row_Air] -> Drag force =1/2*row_a*Cd*Af*v2/2
  Drag force =1/2*row_a*Cd*Af*v2/1 -> Drag Power/1  "Drag_Force (N)"
  [V_at_Wheel] -> Sum/1
  Sum/1 -> drag_v1/1
  [Wind_Speed] -> Sum/2
  drag_v1/1 -> Drag force =1/2*row_a*Cd*Af*v2/4

== system SimBAlink_CL/Road Load & Test Conditions/Vehicle Loads/Grade Force ==
  Display : Display
      settings: Decimation=5
  Fcn : Fcn  Expr=sin(u)
  Grade Force = M*g*sin(road_grade) : Product  Inputs=3  RndMeth=Zero
  d to rad : Gain  Gain=pi/180
  gravity : Constant  Value=9.81
  Drag Power : Outport
  wires:
  Grade Force = M*g*sin(road_grade)/1 -> Display/1, Drag Power/1  "Grade_Force(N)"
  Fcn/1 -> Grade Force = M*g*sin(road_grade)/3
  d to rad/1 -> Fcn/1
  [M] -> Grade Force = M*g*sin(road_grade)/1
  gravity/1 -> Grade Force = M*g*sin(road_grade)/2
  [Road_Grade] -> d to rad/1

== system SimBAlink_CL/Road Load & Test Conditions/Vehicle Loads/Roll Force ==
  Display : Display
      settings: Decimation=5
  Display1 : Display
  Display3 : Display
      settings: Decimation=5
  Fcn : Fcn  Expr=cos(u)
  Fcn1 : Fcn  Expr=0.0048*(9/u(1))^0.5*(400/u(2))^0.25
  Mux : Mux  Inputs=2
  Roll_Force = Cr*M*g*cosd(road_grade) : Product  Inputs=4  RndMeth=Zero
  d to rad : Gain  Gain=pi/180
  "gravity accel (m/s^2) " : Constant  Value=9.81
  Power_roll : Outport
  wires:
  Roll_Force = Cr*M*g*cosd(road_grade)/1 -> Power_roll/1  "Roll_Force (N)"
  d to rad/1 -> Fcn/1
  Fcn/1 -> Roll_Force = Cr*M*g*cosd(road_grade)/4
  [Road_Grade] -> d to rad/1
  [M] -> Mux/2, Display3/1, Roll_Force = Cr*M*g*cosd(road_grade)/2
  Mux/1 -> Fcn1/1
  [Fr_Wheel_Radius] -> Mux/1
  Fcn1/1 -> Roll_Force = Cr*M*g*cosd(road_grade)/1, Display/1  "Cr"
  [Cr] -> Display1/1
  "gravity accel (m/s^2) "/1 -> Roll_Force = Cr*M*g*cosd(road_grade)/3

== system SimBAlink_CL/Vehicle Parameters/Battery Pack/Battery Parameters Calculation ==
  note: if I<0 --> CHARGE
  note: if I>0 --> DISCHARGE
  current1 : Inport
  Demux : Demux  Outputs=3
  OCV Calculation for Battery : Subsystem
      mask Display:
      | color('blue');
      | fprintf('OCV Calculation')
  "R0, C1, R1 Calculation for Battery" : Subsystem
      mask Display:
      | color('blue');
      | fprintf('R0, C1, R1, Calculation', 17)
  SOC Calculation for Battery : Subsystem
      mask Display:
      | color('blue');
      | fprintf('SOC Calculation')
  Switch CHARGE OR DISCHARGE : Switch  Criteria=u2 > Threshold
  tag scope: C1=global, R0=global, R1=global
  wires:
  Demux/3 -> [C1]
  Demux/2 -> [R1]
  Demux/1 -> [R0]
  Switch CHARGE OR DISCHARGE/1 -> Demux/1
  [BAT_Ch] -> Switch CHARGE OR DISCHARGE/3
  [BAT_DisCh] -> Switch CHARGE OR DISCHARGE/1
  current1/1 -> Switch CHARGE OR DISCHARGE/2, SOC Calculation for Battery/1(In1)

== system SimBAlink_CL/Vehicle Parameters/Battery Pack/Battery to Cell ==
  In1 : Inport
  Divide : Product  Inputs=*/
  Out1 : Outport
  tag scope: I_Cell_Request=global
  wires:
  In1/1 -> Divide/1  "I_Bat_Req"
  [cellParallelCount] -> Divide/2
  Divide/1 -> [I_Cell_Request], Out1/1  "I_Cell_Req"

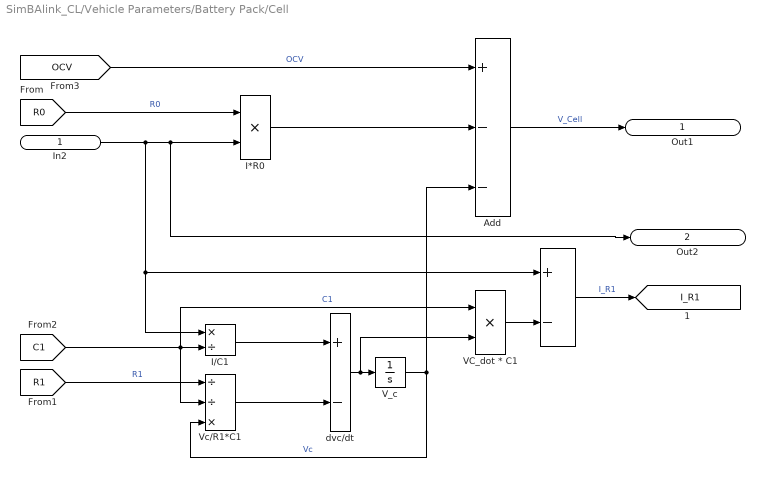
== system SimBAlink_CL/Vehicle Parameters/Battery Pack/Cell ==
  In2 : Inport
  " " : Sum  Inputs=+-
  Add : Sum  Inputs=+--
  I*R0 : Product  RndMeth=Zero
  I/C1 : Product  Inputs=*/
  "VC_dot * C1 " : Product  RndMeth=Zero
  V_c : Integrator
  Vc/R1*C1 : Product  Inputs=//*
  dvc/dt : Sum  Inputs=+-
  Out1 : Outport
  Out2 : Outport  Port=2
  tag scope: I_R1=global
  wires:
  I*R0/1 -> Add/2
  [R0] -> I*R0/1  "R0"
  [OCV] -> Add/1  "OCV"
  In2/1 -> I/C1/1, " "/1, Out2/1, I*R0/2
  Add/1 -> Out1/1  "V_Cell"
  dvc/dt/1 -> "VC_dot * C1 "/2, V_c/1
  I/C1/1 -> dvc/dt/1
  [C1] -> I/C1/2, Vc/R1*C1/2, "VC_dot * C1 "/1  "C1"
  V_c/1 -> Vc/R1*C1/3, Add/3  "Vc"
  Vc/R1*C1/1 -> dvc/dt/2
  [R1] -> Vc/R1*C1/1  "R1"
  "VC_dot * C1 "/1 -> " "/2
  " "/1 -> [I_R1]  "I_R1"

== system SimBAlink_CL/Vehicle Parameters/Battery Pack/Cell to Batt ==
  In1 : Inport
  In2 : Inport  Port=2
  multiply1 : Product  Inputs=**
  multiply2 : Product  Inputs=**
  multiply3 : Product  Inputs=**
  Out1 : Outport
  Out3 : Outport  Port=2
  tag scope: I_Batt=global, V_Batt=global
  wires:
  [cellSeriesCount] -> multiply1/1
  multiply1/1 -> [V_Batt], Out1/1, multiply3/1  "V_Batt"
  In1/1 -> multiply1/2
  In2/1 -> multiply2/1
  [cellParallelCount] -> multiply2/2
  multiply2/1 -> multiply3/2, [I_Batt]  "I_Batt"
  multiply3/1 -> Out3/1  "P_Batt"

== system SimBAlink_CL/Vehicle Parameters/Battery Pack/Thermal Dynamics ==
  " 1" : Sum  Inputs=+-
  " 2" : Sum  Inputs=-+
  A : Constant  Value=BATT_THERMAL.A
  Integrator : Integrator  InitialConditionSource=external  InitialCondition=ambTemp_K
  Pack Heat Generation : Subsystem
  Product : Product  Inputs=3  RndMeth=Zero
  Product1 : Product  RndMeth=Zero
  h : Constant  Value=BATT_THERMAL.h
  m * c : Constant  Value=1/(BATT_THERMAL.cell_mass_g*BATT_THERMAL.c)
  tag scope: T_Batt=global
  wires:
  Pack Heat Generation/1(Out1) -> " 1"/1
  [ambTemp_K] -> " 2"/1
  Integrator/1 -> [T_Batt], " 2"/2  "T_Batt"
  Product/1 -> " 1"/2
  A/1 -> Product/2
  h/1 -> Product/1
  " 2"/1 -> Product/3
  " 1"/1 -> Product1/1
  m * c/1 -> Product1/2
  Product1/1 -> Integrator/1
  [ambTemp_K] -> Integrator/2

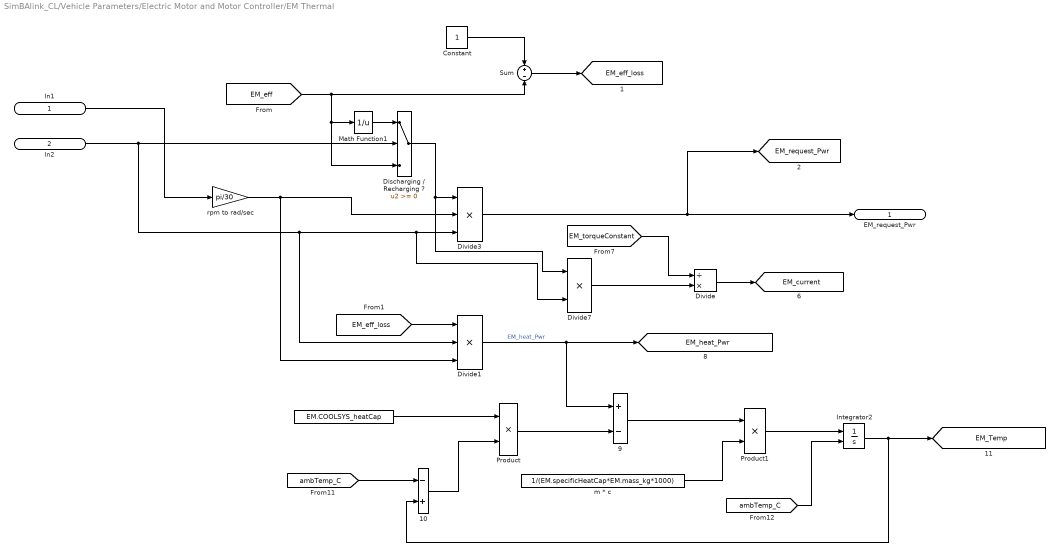
== system SimBAlink_CL/Vehicle Parameters/Electric Motor and Motor Controller/EM Thermal ==
  In1 : Inport
  In2 : Inport  Port=2
  " " : Constant  Value=EM.COOLSYS_heatCap
  " 10" : Sum  Inputs=-+
  " 9" : Sum  Inputs=+-
  Constant : Constant
  Discharging / Recharging ? : Switch  SaturateOnIntegerOverflow=on  InputSameDT=on
  Divide : Product  Inputs=/*
  Divide1 : Product  Inputs=***
  Divide3 : Product  Inputs=***
  Divide7 : Product  Inputs=**
  Integrator2 : Integrator  InitialConditionSource=external  InitialCondition=20
  Math Function1 : Math  Operator=reciprocal  SaturateOnIntegerOverflow=on
  Product : Product  RndMeth=Zero
  Product1 : Product  RndMeth=Zero
  Sum : Sum  Inputs=+-
  m * c : Constant  Value=1/(EM.specificHeatCap*EM.mass_kg*1000)
  rpm to rad/sec : Gain  Gain=pi/30
  EM_request_Pwr : Outport
  tag scope: EM_Temp=global, EM_current=global, EM_eff_loss=global, EM_heat_Pwr=global, EM_request_Pwr=global
  wires:
  In2/1 -> Discharging / Recharging ?/2, Divide1/2, Divide7/2, Divide3/3
  Discharging / Recharging ?/1 -> Divide7/1, Divide3/1
  In1/1 -> rpm to rad/sec/1
  [EM_eff] -> Sum/2, Discharging / Recharging ?/3, Math Function1/1
  Math Function1/1 -> Discharging / Recharging ?/1
  rpm to rad/sec/1 -> Divide3/2, Divide1/3
  Sum/1 -> [EM_eff_loss]
  Constant/1 -> Sum/1
  [EM_eff_loss] -> Divide1/1
  Divide3/1 -> [EM_request_Pwr], EM_request_Pwr/1
  Divide/1 -> [EM_current]
  [EM_torqueConstant] -> Divide/1
  Divide7/1 -> Divide/2
  " 9"/1 -> Product1/1
  Divide1/1 -> [EM_heat_Pwr], " 9"/1  "EM_heat_Pwr"
  " 10"/1 -> Product/2
  Product/1 -> " 9"/2
  m * c/1 -> Product1/2
  Integrator2/1 -> " 10"/2, [EM_Temp]
  " "/1 -> Product/1
  [ambTemp_C] -> Integrator2/2
  Product1/1 -> Integrator2/1
  [ambTemp_C] -> " 10"/1

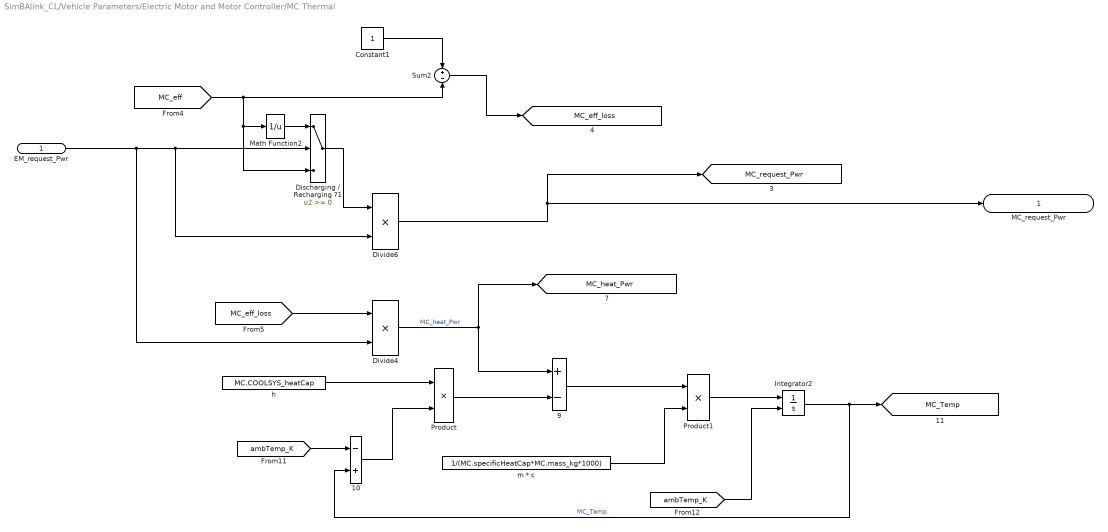
== system SimBAlink_CL/Vehicle Parameters/Electric Motor and Motor Controller/MC Thermal ==
  EM_request_Pwr : Inport
  " 10" : Sum  Inputs=-+
  " 9" : Sum  Inputs=+-
  Constant1 : Constant
  Discharging / Recharging ?1 : Switch  SaturateOnIntegerOverflow=on  InputSameDT=on
  Divide4 : Product  Inputs=**
  Divide6 : Product  Inputs=**
  Integrator2 : Integrator  InitialConditionSource=external  InitialCondition=20
  Math Function2 : Math  Operator=reciprocal  SaturateOnIntegerOverflow=on
  Product : Product  RndMeth=Zero
  Product1 : Product  RndMeth=Zero
  Sum2 : Sum  Inputs=+-
  h : Constant  Value=MC.COOLSYS_heatCap
  m * c : Constant  Value=1/(MC.specificHeatCap*MC.mass_kg*1000)
  MC_request_Pwr : Outport
  tag scope: MC_Temp=global, MC_eff_loss=global, MC_heat_Pwr=global, MC_request_Pwr=global
  wires:
  [MC_eff] -> Sum2/2, Discharging / Recharging ?1/3, Math Function2/1
  Constant1/1 -> Sum2/1
  Divide6/1 -> MC_request_Pwr/1, [MC_request_Pwr]
  Sum2/1 -> [MC_eff_loss]
  Math Function2/1 -> Discharging / Recharging ?1/1
  [MC_eff_loss] -> Divide4/1
  EM_request_Pwr/1 -> Divide4/2, Divide6/2, Discharging / Recharging ?1/2
  Discharging / Recharging ?1/1 -> Divide6/1
  h/1 -> Product/1
  Integrator2/1 -> " 10"/2, [MC_Temp]  "MC_Temp"
  Product/1 -> " 9"/2
  Product1/1 -> Integrator2/1
  [ambTemp_K] -> " 10"/1
  Divide4/1 -> " 9"/1, [MC_heat_Pwr]  "MC_heat_Pwr"
  " 10"/1 -> Product/2
  " 9"/1 -> Product1/1
  m * c/1 -> Product1/2
  [ambTemp_K] -> Integrator2/2

== system SimBAlink_CL/Vehicle Parameters/Powertrain Controller/Braking Strategy ==
  In1 : Inport
  Abs1 : Abs
  Braking Strategy : Stateflow chart  TreatAsAtomicUnit=on
  Gain1 : Gain  Gain=-1
  Out4 : Outport
  Out2 : Outport  Port=2
  Out3 : Outport  Port=3
  wires:
  In1/1 -> Braking Strategy/1(Brake)
  Braking Strategy/2(Front_Wheels_Brake_Request) -> Out3/1  "Front_Wheels_Brake_Request"
  Braking Strategy/1(Rear_Wheels_Brake_Request) -> Out2/1  "Rear_Wheels_Brake_Request"
  [T_Max_Neg_From_EM] -> Abs1/1
  Abs1/1 -> Braking Strategy/3(T_Max_Neg_From_REM)
  Braking Strategy/3(REM_Brake_Torque_Request) -> Gain1/1
  Gain1/1 -> Out4/1  "REM_Brake_Torque_Request"
  [regenPct] -> Braking Strategy/2(data)

== system SimBAlink_CL/Vehicle Parameters/Powertrain Controller/Traction Torque Strategy ==
  In1 : Inport
  Product : Product
  REM_Torque_Request : Outport
  wires:
  Product/1 -> REM_Torque_Request/1  "REM_Torque_Request"
  [T_Max_Pos_From_EM] -> Product/2
  In1/1 -> Product/1

== system SimBAlink_CL/Vehicle Parameters/Battery Pack/Battery Parameters Calculation/OCV Calculation for Battery ==
  SoC vs. OCV : Lookup  InputValues=BATT_OCV.SoC  Table=BATT_OCV.OCV  LookUpMeth=Interpolation-Use End Values
  tag scope: OCV=global
  wires:
  [SOC_Batt] -> SoC vs. OCV/1
  SoC vs. OCV/1 -> [OCV]

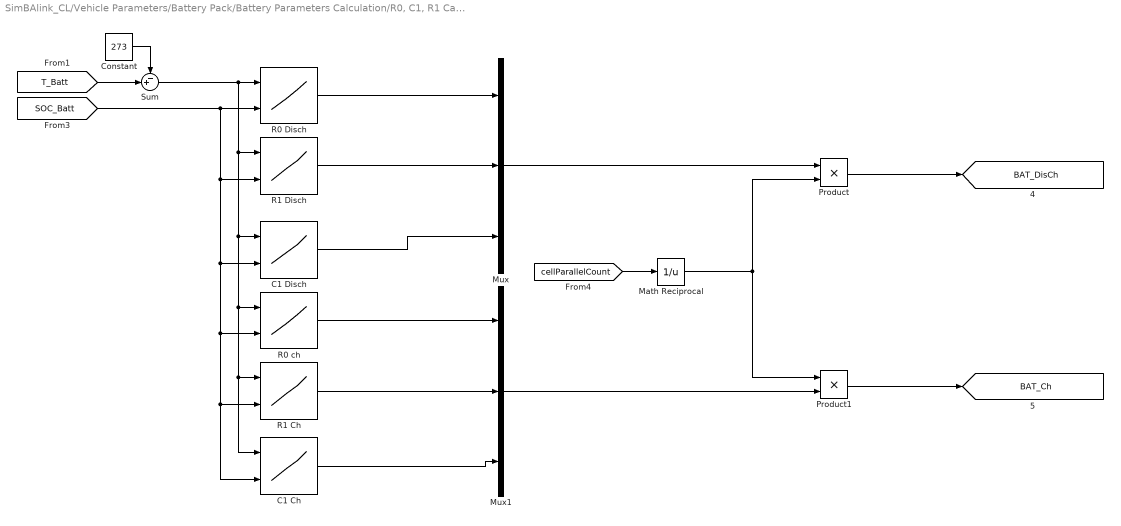
== system SimBAlink_CL/Vehicle Parameters/Battery Pack/Battery Parameters Calculation/R0, C1, R1 Calculation for Battery ==
  C1 Ch : Lookup2D  RowIndex=BATT_ELEC.temp_part  ColumnIndex=BATT_ELEC.soc_part  Table=BATT_ELEC.C1c  LookUpMeth=Interpolation-Use End Values
  C1 Disch : Lookup2D  RowIndex=BATT_ELEC.temp_part  ColumnIndex=BATT_ELEC.soc_part  Table=BATT_ELEC.C1d  LookUpMeth=Interpolation-Use End Values
  Constant : Constant  Value=273
  Math Reciprocal : Math  Operator=reciprocal  SaturateOnIntegerOverflow=on
  Mux : Mux  Inputs=3
  Mux1 : Mux  Inputs=3
  Product : Product
  Product1 : Product
  R0 Disch : Lookup2D  RowIndex=BATT_ELEC.temp_part  ColumnIndex=BATT_ELEC.soc_part  Table=BATT_ELEC.R0d  LookUpMeth=Interpolation-Use End Values
  R0 ch : Lookup2D  RowIndex=BATT_ELEC.temp_part  ColumnIndex=BATT_ELEC.soc_part  Table=BATT_ELEC.R0c  LookUpMeth=Interpolation-Use End Values
  R1 Ch : Lookup2D  RowIndex=BATT_ELEC.temp_part  ColumnIndex=BATT_ELEC.soc_part  Table=BATT_ELEC.R1c  LookUpMeth=Interpolation-Use End Values
  R1 Disch : Lookup2D  RowIndex=BATT_ELEC.temp_part  ColumnIndex=BATT_ELEC.soc_part  Table=BATT_ELEC.R1d  LookUpMeth=Interpolation-Use End Values
  Sum : Sum  Inputs=-+|
  tag scope: BAT_Ch=global, BAT_DisCh=global
  wires:
  Sum/1 -> C1 Ch/1, R1 Ch/1, R0 ch/1, C1 Disch/1, R1 Disch/1, R0 Disch/1
  [SOC_Batt] -> C1 Ch/2, R1 Ch/2, R0 ch/2, C1 Disch/2, R1 Disch/2, R0 Disch/2
  Mux1/1 -> Product1/2
  Constant/1 -> Sum/1
  [T_Batt] -> Sum/2
  R0 Disch/1 -> Mux/1
  C1 Disch/1 -> Mux/3
  R1 Disch/1 -> Mux/2
  R0 ch/1 -> Mux1/1
  R1 Ch/1 -> Mux1/2
  C1 Ch/1 -> Mux1/3
  Product/1 -> [BAT_DisCh]
  Mux/1 -> Product/1
  [cellParallelCount] -> Math Reciprocal/1
  Math Reciprocal/1 -> Product/2, Product1/1
  Product1/1 -> [BAT_Ch]

== system SimBAlink_CL/Vehicle Parameters/Battery Pack/Battery Parameters Calculation/SOC Calculation for Battery ==
  In1 : Inport
  Integrator : Integrator  InitialConditionSource=external  InitialCondition=soc0  LimitOutput=on  UpperSaturationLimit=100  LowerSaturationLimit=0
  Math Reciprocal : Math  Operator=reciprocal  SaturateOnIntegerOverflow=on
  Product1 : Product  Inputs=3  RndMeth=Zero
  Product2 : Product  RndMeth=Zero
  SoC % : Gain  Gain=100
  capacity : Constant  Value=-1/(3600)
  tag scope: SOC_Batt=global
  wires:
  Product1/1 -> SoC %/1
  capacity/1 -> Product1/1
  Math Reciprocal/1 -> Product1/3
  In1/1 -> Product1/2
  Integrator/1 -> [SOC_Batt]  "SoC_Batt"
  SoC %/1 -> Integrator/1
  [soc0] -> Integrator/2
  [cellCapacity] -> Product2/1
  [cellParallelCount] -> Product2/2
  Product2/1 -> Math Reciprocal/1

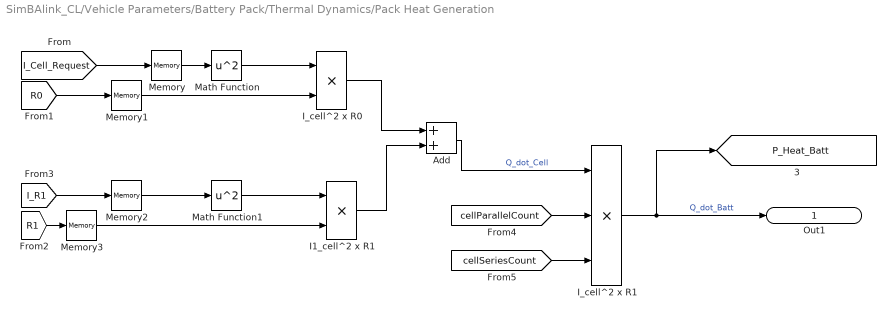
== system SimBAlink_CL/Vehicle Parameters/Battery Pack/Thermal Dynamics/Pack Heat Generation ==
  Add : Sum
  I1_cell^2 x R1 : Product  RndMeth=Zero
  I_cell^2 x R0 : Product  RndMeth=Zero
  I_cell^2 x R1 : Product  Inputs=3  RndMeth=Zero
  Math Function : Math  Operator=square  SaturateOnIntegerOverflow=on
  Math Function1 : Math  Operator=square  SaturateOnIntegerOverflow=on
  Memory{,1..3} (4 alike) : Memory
  Out1 : Outport
  tag scope: P_Heat_Batt=global
  wires:
  [R0] -> Memory1/1
  [I_Cell_Request] -> Memory/1
  Math Function/1 -> I_cell^2 x R0/1
  [I_R1] -> Memory2/1
  [R1] -> Memory3/1
  I1_cell^2 x R1/1 -> Add/2
  I_cell^2 x R0/1 -> Add/1
  Add/1 -> I_cell^2 x R1/1  "Q_dot_Cell"
  I_cell^2 x R1/1 -> [P_Heat_Batt], Out1/1  "Q_dot_Batt"
  [cellParallelCount] -> I_cell^2 x R1/2
  [cellSeriesCount] -> I_cell^2 x R1/3
  Math Function1/1 -> I1_cell^2 x R1/1
  Memory/1 -> Math Function/1
  Memory1/1 -> I_cell^2 x R0/2
  Memory2/1 -> Math Function1/1
  Memory3/1 -> I1_cell^2 x R1/2

== stateflow chart SimBAlink_CL/Vehicle Parameters/Powertrain Controller/Braking Strategy/Braking Strategy ==
  state No_Brake
    during:
    Front_Wheels_Brake_Request=0;
    Rear_Wheels_Brake_Request=0;
    REM_Brake_Torque_Request=0;
  state Normal_Brake
    during:
    Front_Wheels_Brake_Request=1*Brake;
    REM_Brake_Torque_Request=0*Brake*T_Max_Neg_From_REM;
    Rear_Wheels_Brake_Request=0*Brake;
  (default) -> No_Brake
  No_Brake -> Normal_Brake : [Brake>0.01]
  Normal_Brake -> No_Brake : [Brake<0.01]
  data: Brake input; data input; Rear_Wheels_Brake_Request output double; Front_Wheels_Brake_Request output double; T_Max_Neg_From_REM input; REM_Brake_Torque_Request output double
